simulink model "differential"  (R2018a)
settings: Solver=VariableStepDiscrete  StartTime=0.0  StopTime=0.15  RelTol=1e-3
undefined symbols (not defined in the file or in its folder): DiscIntNeverNeededParam
libraries: powerlib x45
settings Model: Creator=user  LastModifiedBy=user

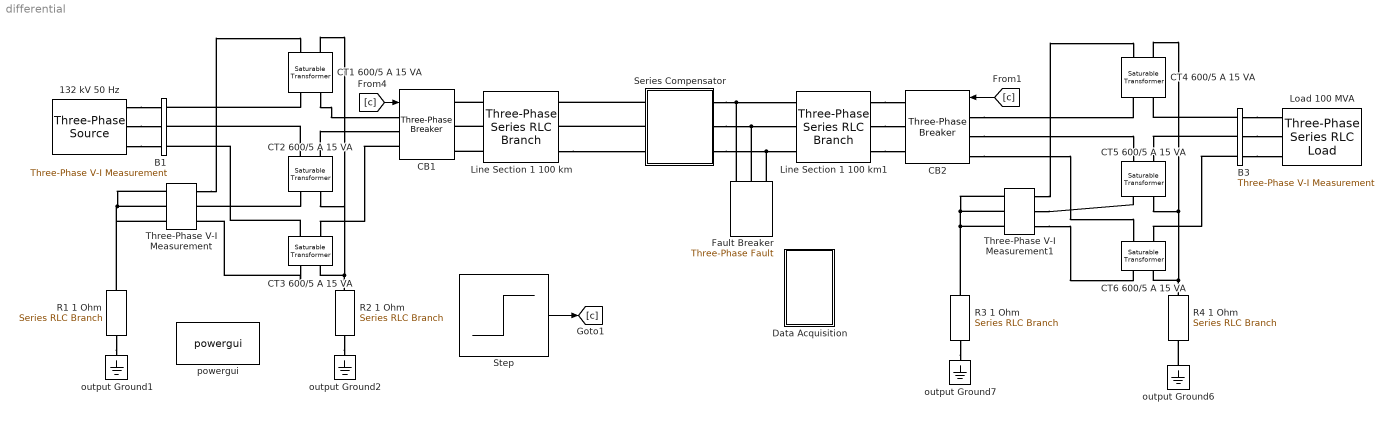
== system differential ==
  132 kV 50 Hz : powerlib/Electrical Sources/Three-Phase Source  InternalConnection=Yg  VoltagePhases=off  Voltage=132e3  PhaseAngle=0  Voltage_phases=[25e3 25e3 25e3]/sqrt(3)  PhaseAngles_phases=[0 -120 +120]  Frequency=50  NonIdealSource=on  SpecifyImpedance=on  Resistance=132^2/30000/10  Inductance=132^2/30000/377  ShortCircuitLevel=1000e6  BaseVoltage=132e3  XRratio=10  BusType=swing  Pref=150e6  Qref=0  Prefabc=[10e3, 10e3, 10e3]  Qrefabc=[0, 0, 0]  Qmin=0  Qmax=5e6
  B1 : powerlib/Measurements/Three-Phase V-I Measurement  VoltageMeasurement=phase-to-phase  SetLabelV=on  LabelV=Vabc_B1  Vpu=off  VpuLL=on  CurrentMeasurement=yes  SetLabelI=on  LabelI=Iabc_B1  Ipu=off  Pbase=100e6  Vbase=132e3  OutputType=Complex  PhasorSimulation=off  PSBequivalent=0
  B3 : powerlib/Measurements/Three-Phase V-I Measurement  VoltageMeasurement=phase-to-phase  SetLabelV=on  LabelV=Vabc_B2  Vpu=off  VpuLL=on  CurrentMeasurement=yes  SetLabelI=on  LabelI=Iabc_B2  Ipu=off  Pbase=100e6  Vbase=132e3  OutputType=Complex  PhasorSimulation=off  PSBequivalent=0
  CB1 : powerlib/Elements/Three-Phase Breaker  InitialState=closed  SwitchA=off  SwitchB=off  SwitchC=off  SwitchTimes=[5/60]  External=on  BreakerResistance=0.001  SnubberResistance=10e6  SnubberCapacitance=inf  Measurements=None
      settings: AttributesFormatString=\n
  CB2 : powerlib/Elements/Three-Phase Breaker  InitialState=closed  SwitchA=off  SwitchB=off  SwitchC=off  SwitchTimes=[5/60]  External=on  BreakerResistance=0.001  SnubberResistance=10e6  SnubberCapacitance=inf  Measurements=None
      settings: AttributesFormatString=\n
  CT1 600/5 A 15 VA : powerlib/Elements/Saturable Transformer  ThreeWindings=off  Hysteresis=off  DataFile='hysteresis'  Measurements=Winding currents  UNITS=pu  NominalPower=[15 50]  Winding1=[5*1/600 0.001 0.04]  Winding2=[5 0.001 0.04]  Winding3=[5 0.001 0.039999]  Saturation=[0 0 ; 0.01 10 ; 1 10.5]  CoreLoss=100  MoreParameters=off  BreakLoop=off  DataType=off  InitialFlux=-9.06091866417811e-08  TransfoNumber=1
      settings: AttributesFormatString=\n  SourceProductName=Simscape Power Systems  SourceProductBaseCode=PS
  CT2 600/5 A 15 VA : powerlib/Elements/Saturable Transformer  ThreeWindings=off  Hysteresis=off  DataFile='hysteresis'  Measurements=Winding currents  UNITS=pu  NominalPower=[15 50]  Winding1=[5*1/600 0.001 0.04]  Winding2=[5 0.001 0.04 ]  Winding3=[5 0.001 0.04 ]  Saturation=[0 0 ; 0.01 10 ; 1 10.5]  CoreLoss=100  MoreParameters=off  BreakLoop=off  DataType=off  InitialFlux=-1.84905677710759e-08  TransfoNumber=1
      settings: AttributesFormatString=\n  SourceProductName=Simscape Power Systems  SourceProductBaseCode=PS
  CT3 600/5 A 15 VA : powerlib/Elements/Saturable Transformer  ThreeWindings=off  Hysteresis=off  DataFile='hysteresis'  Measurements=Winding currents  UNITS=pu  NominalPower=[15 50]  Winding1=[5*1/600 0.001 0.04]  Winding2=[5 0.001 0.04]  Winding3=[5 0.001 0.039999]  Saturation=[0 0 ; 0.01 10 ; 1 10.5]  CoreLoss=100  MoreParameters=off  BreakLoop=off  DataType=off  InitialFlux=1.09099754414671e-07  TransfoNumber=1
      settings: AttributesFormatString=\n  SourceProductName=Simscape Power Systems  SourceProductBaseCode=PS
  CT4 600/5 A 15 VA : powerlib/Elements/Saturable Transformer  ThreeWindings=off  Hysteresis=off  DataFile='hysteresis'  Measurements=Winding currents  UNITS=pu  NominalPower=[15 50]  Winding1=[5*1/600 0.001 0.04]  Winding2=[5 0.001 0.04]  Winding3=[5 0.001 0.039999]  Saturation=[0 0 ; 0.01 10 ; 1 10.5]  CoreLoss=100  MoreParameters=off  BreakLoop=off  DataType=off  InitialFlux=-9.06015492379664e-08  TransfoNumber=1
      settings: AttributesFormatString=\n  SourceProductName=Simscape Power Systems  SourceProductBaseCode=PS
  CT5 600/5 A 15 VA : powerlib/Elements/Saturable Transformer  ThreeWindings=off  Hysteresis=off  DataFile='hysteresis'  Measurements=Winding currents  UNITS=pu  NominalPower=[15 50]  Winding1=[5*1/600 0.001 0.04]  Winding2=[5 0.001 0.04 ]  Winding3=[5 0.001 0.04 ]  Saturation=[0 0 ; 0.01 10 ; 1 10.5]  CoreLoss=100  MoreParameters=off  BreakLoop=off  DataType=off  InitialFlux=-1.84519480177304e-08  TransfoNumber=1
      settings: AttributesFormatString=\n  SourceProductName=Simscape Power Systems  SourceProductBaseCode=PS
  CT6 600/5 A 15 VA : powerlib/Elements/Saturable Transformer  ThreeWindings=off  Hysteresis=off  DataFile='hysteresis'  Measurements=Winding currents  UNITS=pu  NominalPower=[15 50]  Winding1=[5*1/600 0.001 0.04]  Winding2=[5 0.001 0.04]  Winding3=[5 0.001 0.039999]  Saturation=[0 0 ; 0.01 10 ; 1 10.5]  CoreLoss=100  MoreParameters=off  BreakLoop=off  DataType=off  InitialFlux=1.09053497257451e-07  TransfoNumber=1
      settings: AttributesFormatString=\n  SourceProductName=Simscape Power Systems  SourceProductBaseCode=PS
  Data Acquisition : Subsystem  mask(Data Acquisition){}
      mask Display: disp('Scopes')
  Fault Breaker : powerlib/Elements/Three-Phase Fault  InitialStates=0  FaultA=on  FaultB=off  FaultC=off  GroundFault=off  SwitchTimes=[2.5/60 ]  External=off  SwitchStatus=NaN  FaultResistance=0.001  GroundResistance=0.01  SnubberResistance=1e6  SnubberCapacitance=inf  Measurements=Fault currents
  Line Section 1 100 km : powerlib/Elements/Three-Phase Series RLC Branch  LConnTagsString=A|B|C  RConnTagsString=A|B|C  BranchType=RL  Resistance=36.7  Inductance=0.462  Capacitance=0.001  Measurements=None
  Line Section 1 100 km1 : powerlib/Elements/Three-Phase Series RLC Branch  LConnTagsString=A|B|C  RConnTagsString=A|B|C  BranchType=RL  Resistance=36.7  Inductance=0.462  Capacitance=0.001  Measurements=None
  Load 100 MVA : powerlib/Elements/Three-Phase Series RLC Load  LConnTagsString=A|B|C  Configuration=Y (grounded)  NominalVoltage=132e3  Vabc=[1e3 1e3 1e3]  Vabcp=[1e3 1e3 1e3]  NominalFrequency=50  UnbalancedPower=off  ActivePower=50e6  InductivePower=25e6  CapacitivePower=0  Pabc=[10e3 9e3 11e3]  QLabc=[100 90 110]  QCabc=[100 90 110]  Pabcp=[10e3 9e3 11e3]  QLabcp=[100 90 110]  QCabcp=[100 90 110]  Measurements=None  LoadType=constant Z
  R1 1 Ohm : powerlib/Elements/Series RLC Branch  LConnTagsString=__new0  RConnTagsString=__new0  BranchType=R  Resistance=1  Inductance=[]  SetiL0=off  InitialCurrent=0  Capacitance=[]  Setx0=off  InitialVoltage=0  Measurements=None
  R2 1 Ohm : powerlib/Elements/Series RLC Branch  LConnTagsString=__new0  RConnTagsString=__new0  BranchType=R  Resistance=1  Inductance=[]  SetiL0=off  InitialCurrent=0  Capacitance=[]  Setx0=off  InitialVoltage=0  Measurements=None
  R3 1 Ohm : powerlib/Elements/Series RLC Branch  LConnTagsString=__new0  RConnTagsString=__new0  BranchType=R  Resistance=1  Inductance=[]  SetiL0=off  InitialCurrent=0  Capacitance=[]  Setx0=off  InitialVoltage=0  Measurements=None
  R4 1 Ohm : powerlib/Elements/Series RLC Branch  LConnTagsString=__new0  RConnTagsString=__new0  BranchType=R  Resistance=1  Inductance=[]  SetiL0=off  InitialCurrent=0  Capacitance=[]  Setx0=off  InitialVoltage=0  Measurements=None
  Series Compensator : Subsystem
      mask Display: plot(0,0,100,100,[25 45],[50 50], [45 45],[35 65],[55 55],[35 65], [55 75],[50 50])
  Step : Step  Time=2/60  Before=1  VectorParams1D=off  ZeroCross=off
  Three-Phase V-I Measurement : powerlib/Measurements/Three-Phase V-I Measurement  VoltageMeasurement=no  SetLabelV=off  LabelV=Vabc  Vpu=off  VpuLL=off  CurrentMeasurement=yes  SetLabelI=on  LabelI=Iabc  Ipu=off  Pbase=100e6  Vbase=500e3  OutputType=Complex  PhasorSimulation=off  PSBequivalent=0
  Three-Phase V-I Measurement1 : powerlib/Measurements/Three-Phase V-I Measurement  VoltageMeasurement=no  SetLabelV=off  LabelV=Vabc  Vpu=off  VpuLL=off  CurrentMeasurement=yes  SetLabelI=on  LabelI=Iabc1  Ipu=off  Pbase=100e6  Vbase=500e3  OutputType=Complex  PhasorSimulation=off  PSBequivalent=0
  output Ground{1..2,6..7} (4 alike) : powerlib/Elements/Ground  LConnTagsString=a
  powergui : powerlib/powergui  Priority=2  SimulationMode=Discrete  SampleTime=50e-6  frequency=60  Iterations=50  frequencyindice=50  Pbase=100e6  ErrMax=0.0001  UnitsV=kV  UnitsW=MW  buscounter=0  FunctionMessages=off  echomessages=off  EnableUseOfTLC=off  CurrentSourceSwitches=off  DisableSnubberDevices=off  DisableRonSwitches=off  DisableVfSwitches=off  DisplayEquations=off  SolverType=Tustin/Backward Euler (TBE)  Interpol=off  ExternalGateDelay=off  methode=off  Ts=100  x0status=blocks  SPID=off  SwTol=0  HookPort=off  RestoreLinks=warning  ResistiveCurrentMeasurement=off  Frange=0:0.5:500  Ylog=off  Xlog=off  ShowGrid=off  save=on  variable=Zmes  structure=0  ZoomFFT=on  StartTime=0.0  cycles=1  DisplayStyle=off  fundamental=60  FreqAxis=off  MaxFrequency=1000  frequencyindicesteady=1  RmsSteady=1  display=off
  wires:
  [c] -> CB1/1
  [c] -> CB2/1
  Step/1 -> [c]
  connections:
  Three-Phase V-I Measurement/RConn2 -- Three-Phase V-I Measurement/RConn1 -- R1 1 Ohm/LConn1 -- Three-Phase V-I Measurement/RConn3
  R2 1 Ohm/LConn1 -- CT1 600/5 A 15 VA/RConn2 -- CT2 600/5 A 15 VA/RConn2 -- CT3 600/5 A 15 VA/RConn2
  Series Compensator/RConn3 -- Line Section 1 100 km1/LConn3 -- Fault Breaker/LConn3
  Series Compensator/RConn2 -- Line Section 1 100 km1/LConn2 -- Fault Breaker/LConn2
  Series Compensator/RConn1 -- Line Section 1 100 km1/LConn1 -- Fault Breaker/LConn1
  R1 1 Ohm/RConn1 -- output Ground1/LConn1
  Line Section 1 100 km/LConn2 -- CB1/RConn2
  CT2 600/5 A 15 VA/RConn1 -- Three-Phase V-I Measurement/LConn2
  CT3 600/5 A 15 VA/RConn1 -- Three-Phase V-I Measurement/LConn3
  Three-Phase V-I Measurement/LConn1 -- CT1 600/5 A 15 VA/RConn1
  CT1 600/5 A 15 VA/LConn2 -- CB1/LConn1
  Line Section 1 100 km/RConn3 -- Series Compensator/LConn3
  CT2 600/5 A 15 VA/LConn1 -- B1/RConn2
  R2 1 Ohm/RConn1 -- output Ground2/LConn1
  Line Section 1 100 km/LConn3 -- CB1/RConn3
  132 kV 50 Hz/RConn1 -- B1/LConn1
  Series Compensator/LConn2 -- Line Section 1 100 km/RConn2
  Series Compensator/LConn1 -- Line Section 1 100 km/RConn1
  CB1/LConn3 -- CT3 600/5 A 15 VA/LConn2
  CT1 600/5 A 15 VA/LConn1 -- B1/RConn1
  132 kV 50 Hz/RConn2 -- B1/LConn2
  Line Section 1 100 km/LConn1 -- CB1/RConn1
  CT3 600/5 A 15 VA/LConn1 -- B1/RConn3
  132 kV 50 Hz/RConn3 -- B1/LConn3
  CT2 600/5 A 15 VA/LConn2 -- CB1/LConn2
  CT5 600/5 A 15 VA/RConn2 -- CT4 600/5 A 15 VA/RConn2 -- R4 1 Ohm/LConn1 -- CT6 600/5 A 15 VA/RConn2
  Three-Phase V-I Measurement1/RConn3 -- R3 1 Ohm/LConn1 -- Three-Phase V-I Measurement1/RConn2 -- Three-Phase V-I Measurement1/RConn1
  B3/RConn3 -- Load 100 MVA/LConn3
  B3/LConn3 -- CT6 600/5 A 15 VA/LConn2
  Line Section 1 100 km1/RConn1 -- CB2/RConn1
  output Ground6/LConn1 -- R4 1 Ohm/RConn1
  Line Section 1 100 km1/RConn2 -- CB2/RConn2
  R3 1 Ohm/RConn1 -- output Ground7/LConn1
  CB2/LConn1 -- CT4 600/5 A 15 VA/LConn1
  CB2/LConn2 -- CT5 600/5 A 15 VA/LConn1
  Three-Phase V-I Measurement1/LConn2 -- CT5 600/5 A 15 VA/RConn1
  Three-Phase V-I Measurement1/LConn1 -- CT4 600/5 A 15 VA/RConn1
  B3/LConn2 -- CT5 600/5 A 15 VA/LConn2
  B3/LConn1 -- CT4 600/5 A 15 VA/LConn2
  CB2/LConn3 -- CT6 600/5 A 15 VA/LConn1
  Line Section 1 100 km1/RConn3 -- CB2/RConn3
  B3/RConn1 -- Load 100 MVA/LConn1
  B3/RConn2 -- Load 100 MVA/LConn2
  Three-Phase V-I Measurement1/LConn3 -- CT6 600/5 A 15 VA/RConn1

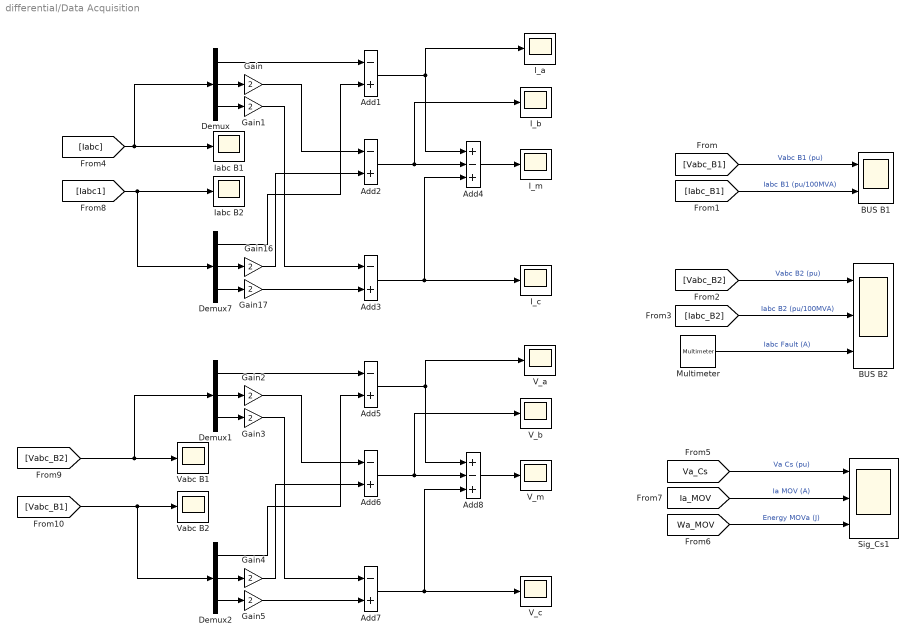
== system differential/Data Acquisition ==
  Add{1..3,5..7} (6 alike) : Sum  Inputs=-+
  Add4 : Sum  Inputs=+-+
  Add8 : Sum  Inputs=+-+
  BUS B1 : Scope  NumInputPorts=2
  BUS B2 : Scope  NumInputPorts=3
  Demux{,1..2,7} (4 alike) : Demux  Outputs=3
  Gain{,1..5,16..17} (8 alike) : Gain  Gain=2
  I_a : Scope
  I_b : Scope
  I_c : Scope
  I_m : Scope
  Iabc B1 : Scope
  Iabc B2 : Scope
  Multimeter : powerlib/Measurements/Multimeter  Tag=PoWeRsYsTeMmEaSuReMeNt  PhasorSimulation=off  OutputType=Magnitude  sel=[1 2 3]  L=15  Gain=[1 1 1]  yselected={'Ib: Fault Breaker/Fault A','Ib: Fault Breaker/Fault B','Ib: Fault Breaker/Fault C'};  PSBOutputType=1  PSBequivalent=0  AxesSetting=[0,0.1,-100,100]  Display=0  SavedBlockNames={}
      settings: AttributesFormatString=\n
  Sig_Cs1 : Scope  NumInputPorts=3
  V_a : Scope
  V_b : Scope
  V_c : Scope
  V_m : Scope
  Vabc B1 : Scope
  Vabc B2 : Scope
  wires:
  [Vabc_B1] -> BUS B1/1  "Vabc B1 (pu)"
  [Iabc_B1] -> BUS B1/2  "Iabc B1 (pu/100MVA)"
  [Vabc_B2] -> BUS B2/1  "Vabc B2 (pu)"
  [Iabc_B2] -> BUS B2/2  "Iabc B2 (pu/100MVA)"
  [Va_Cs] -> Sig_Cs1/1  "Va Cs (pu)"
  [Ia_MOV] -> Sig_Cs1/2  "Ia MOV (A)"
  [Wa_MOV] -> Sig_Cs1/3  "Energy MOVa (J)"
  Multimeter/1 -> BUS B2/3  "Iabc Fault (A)"
  Gain/1 -> Add2/1
  Demux/3 -> Gain1/1
  Demux/2 -> Gain/1
  Gain1/1 -> Add3/1
  [Iabc] -> Iabc B1/1, Demux/1
  [Iabc1] -> Iabc B2/1, Demux7/1
  Gain17/1 -> Add3/2
  Demux7/3 -> Gain17/1
  Demux7/1 -> Add1/2
  Demux7/2 -> Gain16/1
  Demux/1 -> Add1/1
  Gain16/1 -> Add2/2
  Add4/1 -> I_m/1
  Add1/1 -> I_a/1, Add4/1
  Add2/1 -> I_b/1, Add4/2
  Add3/1 -> Add4/3, I_c/1
  Demux2/3 -> Gain5/1
  Demux1/1 -> Add5/1
  [Vabc_B1] -> Vabc B2/1, Demux2/1
  [Vabc_B2] -> Vabc B1/1, Demux1/1
  Add8/1 -> V_m/1
  Gain4/1 -> Add6/2
  Gain2/1 -> Add6/1
  Gain5/1 -> Add7/2
  Add6/1 -> V_b/1, Add8/2
  Demux1/3 -> Gain3/1
  Demux1/2 -> Gain2/1
  Demux2/1 -> Add5/2
  Gain3/1 -> Add7/1
  Add5/1 -> V_a/1, Add8/1
  Demux2/2 -> Gain4/1
  Add7/1 -> Add8/3, V_c/1

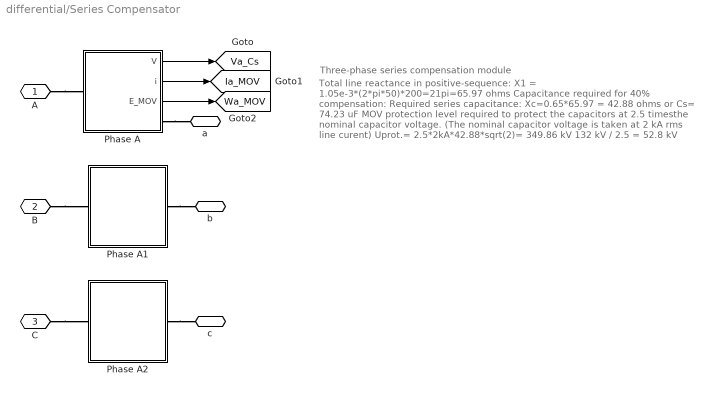
== system differential/Series Compensator ==
  note: Three-phase series compensation module
  note: Total line reactance in positive-sequence:
      |  X1 = 1.05e-3*(2*pi*50)*200=21pi=65.97 ohms
      |
      | Capacitance required for 40% compensation:
      |
      | Required series capacitance:
      | Xc=0.65*65.97 = 42.88 ohms
      | or Cs= 74.23 uF
      |
      | MOV protection level required to protect the capacitors
      | at 2.5 timesthe nominal capacitor voltage.
      | (The nominal capacitor voltage is taken at 2 kA  rms line curent)
      |
      | Uprot.= 2.5*2kA*42.88*sqrt(2)= 349.86 kV
      |
      | 132 kV / 2.5 = 52.8 kV
  Phase A : Subsystem
  Phase A1 : Subsystem
  Phase A2 : Subsystem
  A : PMIOPort  Side=Left
  B : PMIOPort  Port=2  Side=Left
  C : PMIOPort  Port=3  Side=Left
  a : PMIOPort  Port=4  Side=Right
  b : PMIOPort  Port=5  Side=Right
  c : PMIOPort  Port=6  Side=Right
  tag scope: Ia_MOV=global, Va_Cs=global, Wa_MOV=global
  wires:
  Phase A/2(i) -> [Ia_MOV]
  Phase A/1(V) -> [Va_Cs]
  Phase A/3(E_MOV) -> [Wa_MOV]
  connections:
  A/RConn1 -- Phase A/LConn1
  B/RConn1 -- Phase A1/LConn1
  C/RConn1 -- Phase A2/LConn1
  Phase A/RConn1 -- a/RConn1
  Phase A1/RConn1 -- b/RConn1
  Phase A2/RConn1 -- c/RConn1

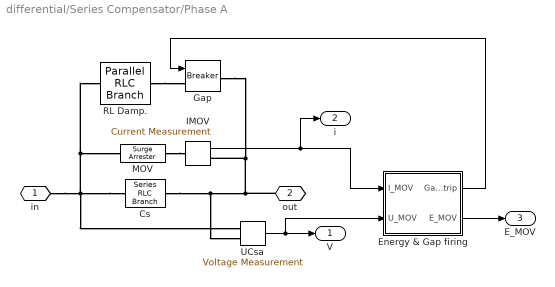
== system differential/Series Compensator/Phase A ==
  Cs : powerlib/Elements/Series RLC Branch  LConnTagsString=__new0  RConnTagsString=__new0  BranchType=C  Resistance=1.0  Inductance=1.0  SetiL0=off  InitialCurrent=0  Capacitance=95e-6  Setx0=off  InitialVoltage=0  Measurements=None
  Energy & Gap firing : Subsystem
  Gap : powerlib/Elements/Breaker  InitialState=0  SwitchingTimes="[ 4/60  5/60 ]"  External=on  BreakerResistance=0.001  SnubberResistance=inf  SnubberCapacitance=0  Measurements=None  MoreParameters=off  NoBreakLoop=off
      settings: AttributesFormatString=\n  SourceProductName=Simscape Power Systems
  IMOV : powerlib/Measurements/Current Measurement  Tag=PoWeRsYsTeMmEaSuReMeNt  PhasorSimulation=off  OutputType=Magnitude  PSBequivalent=0
  MOV : powerlib/Elements/Surge Arrester  ProtectionVoltage=54e+03  Columns=27  ReferenceCurrent=200  Segment1=[.955 50]  Segment2=[1.0 25]  Segment3=[.9915 16.5]  Measurements=None  BreakLoop=on
      settings: AttributesFormatString=\n  SourceProductName=Simscape Power Systems  SourceProductBaseCode=PS
  RL Damp. : powerlib/Elements/Parallel RLC Branch  LConnTagsString=a  RConnTagsString=__new0  BranchType=RL  Resistance=7.5  Inductance=1.7e-3  SetiL0=off  InitialCurrent=0  Capacitance=1.0  Setx0=off  InitialVoltage=0  Measurements=None
  UCsa : powerlib/Measurements/Voltage Measurement  Tag=PoWeRsYsTeMmEaSuReMeNt  PhasorSimulation=off  OutputType=Magnitude  PSBequivalent=0
  in : PMIOPort  Side=Left
  "out " : PMIOPort  Port=2  Side=Right
  V : Outport
  i : Outport  Port=2
  E_MOV : Outport  Port=3
  wires:
  Energy & Gap firing/2(E_MOV) -> E_MOV/1
  IMOV/1 -> Energy & Gap firing/1(I_MOV), i/1
  UCsa/1 -> Energy & Gap firing/2(U_MOV), V/1
  Energy & Gap firing/1(Gap_trip) -> Gap/1
  connections:
  MOV/RConn1 -- IMOV/LConn1
  Cs/LConn1 -- UCsa/LConn1 -- in/RConn1 -- RL Damp./LConn1 -- MOV/LConn1
  RL Damp./RConn1 -- Gap/LConn1
  Cs/RConn1 -- "out "/RConn1 -- IMOV/RConn1 -- Gap/RConn1 -- UCsa/LConn2

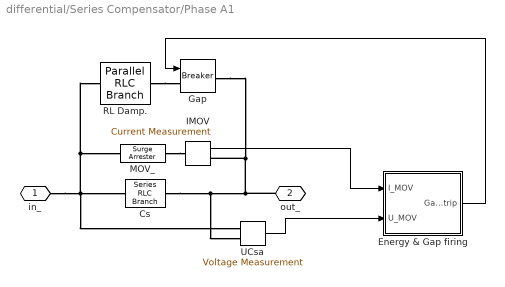
== system differential/Series Compensator/Phase A1 ==
  Cs : powerlib/Elements/Series RLC Branch  LConnTagsString=__new0  RConnTagsString=__new0  BranchType=C  Resistance=1.0  Inductance=1.0  SetiL0=off  InitialCurrent=0  Capacitance=95e-6  Setx0=off  InitialVoltage=0  Measurements=None
  Energy & Gap firing : Subsystem
  Gap : powerlib/Elements/Breaker  InitialState=0  SwitchingTimes="[ 4/60  5/60 ]"  External=on  BreakerResistance=0.001  SnubberResistance=inf  SnubberCapacitance=0  Measurements=None  MoreParameters=off  NoBreakLoop=off
      settings: AttributesFormatString=\n  SourceProductName=Simscape Power Systems
  IMOV : powerlib/Measurements/Current Measurement  Tag=PoWeRsYsTeMmEaSuReMeNt  PhasorSimulation=off  OutputType=Magnitude  PSBequivalent=0
  MOV_ : powerlib/Elements/Surge Arrester  ProtectionVoltage=54e+03  Columns=27  ReferenceCurrent=200  Segment1=[.955 50]  Segment2=[1.0 25]  Segment3=[.9915 16.5]  Measurements=None  BreakLoop=on
      settings: AttributesFormatString=\n  SourceProductName=Simscape Power Systems  SourceProductBaseCode=PS
  RL Damp. : powerlib/Elements/Parallel RLC Branch  LConnTagsString=a  RConnTagsString=__new0  BranchType=RL  Resistance=7.5  Inductance=1.7e-3  SetiL0=off  InitialCurrent=0  Capacitance=1.0  Setx0=off  InitialVoltage=0  Measurements=None
  UCsa : powerlib/Measurements/Voltage Measurement  Tag=PoWeRsYsTeMmEaSuReMeNt  PhasorSimulation=off  OutputType=Magnitude  PSBequivalent=0
  in_ : PMIOPort  Side=Left
  "out_ " : PMIOPort  Port=2  Side=Right
  wires:
  Energy & Gap firing/1(Gap_trip) -> Gap/1
  UCsa/1 -> Energy & Gap firing/2(U_MOV)
  IMOV/1 -> Energy & Gap firing/1(I_MOV)
  connections:
  "out_ "/RConn1 -- UCsa/LConn2 -- Cs/RConn1 -- Gap/RConn1 -- IMOV/RConn1
  RL Damp./RConn1 -- Gap/LConn1
  in_/RConn1 -- UCsa/LConn1 -- Cs/LConn1 -- MOV_/LConn1 -- RL Damp./LConn1
  MOV_/RConn1 -- IMOV/LConn1

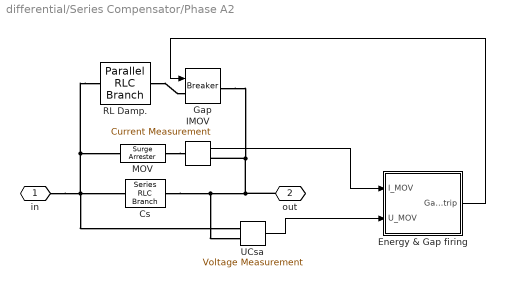
== system differential/Series Compensator/Phase A2 ==
  Cs : powerlib/Elements/Series RLC Branch  LConnTagsString=__new0  RConnTagsString=__new0  BranchType=C  Resistance=1.0  Inductance=1.0  SetiL0=off  InitialCurrent=0  Capacitance=95e-6  Setx0=off  InitialVoltage=0  Measurements=None
  Energy & Gap firing : Subsystem
  Gap : powerlib/Elements/Breaker  InitialState=0  SwitchingTimes="[ 4/60  5/60 ]"  External=on  BreakerResistance=0.001  SnubberResistance=inf  SnubberCapacitance=0  Measurements=None  MoreParameters=off  NoBreakLoop=off
      settings: AttributesFormatString=\n  SourceProductName=Simscape Power Systems
  IMOV : powerlib/Measurements/Current Measurement  Tag=PoWeRsYsTeMmEaSuReMeNt  PhasorSimulation=off  OutputType=Magnitude  PSBequivalent=0
  MOV : powerlib/Elements/Surge Arrester  ProtectionVoltage=54e+03  Columns=27  ReferenceCurrent=200  Segment1=[.955 50]  Segment2=[1.0 25]  Segment3=[.9915 16.5]  Measurements=None  BreakLoop=on
      settings: AttributesFormatString=\n  SourceProductName=Simscape Power Systems  SourceProductBaseCode=PS
  RL Damp. : powerlib/Elements/Parallel RLC Branch  LConnTagsString=a  RConnTagsString=__new0  BranchType=RL  Resistance=7.5  Inductance=1.7e-3  SetiL0=off  InitialCurrent=0  Capacitance=1.0  Setx0=off  InitialVoltage=0  Measurements=None
  UCsa : powerlib/Measurements/Voltage Measurement  Tag=PoWeRsYsTeMmEaSuReMeNt  PhasorSimulation=off  OutputType=Magnitude  PSBequivalent=0
  in : PMIOPort  Side=Left
  "out " : PMIOPort  Port=2  Side=Right
  wires:
  IMOV/1 -> Energy & Gap firing/1(I_MOV)
  UCsa/1 -> Energy & Gap firing/2(U_MOV)
  Energy & Gap firing/1(Gap_trip) -> Gap/1
  connections:
  MOV/RConn1 -- IMOV/LConn1
  RL Damp./LConn1 -- MOV/LConn1 -- Cs/LConn1 -- UCsa/LConn1 -- in/RConn1
  RL Damp./RConn1 -- Gap/LConn1
  IMOV/RConn1 -- Gap/RConn1 -- Cs/RConn1 -- UCsa/LConn2 -- "out "/RConn1

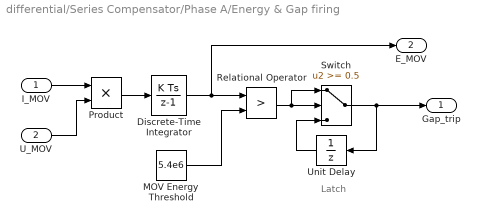
== system differential/Series Compensator/Phase A/Energy & Gap firing ==
  note: Latch
  I_MOV : Inport
  U_MOV : Inport  Port=2
  Discrete-Time Integrator : DiscreteIntegrator  SampleTime=-1  ICPrevOutput=DiscIntNeverNeededParam  ICPrevScaledInput=DiscIntNeverNeededParam
  MOV Energy Threshold : Constant  Value=5.4e6
  Product : Product  SaturateOnIntegerOverflow=on  InputSameDT=on  OutDataTypeStr=Inherit: Same as first input
  Relational Operator : RelationalOperator  Operator=>  ZeroCross=off  RndMeth=Nearest  InputSameDT=on
  Switch : Switch  Threshold=0.5  ZeroCross=off  InputSameDT=on
  Unit Delay : UnitDelay  SampleTime=-1
  Gap_trip : Outport
  E_MOV : Outport  Port=2  InitialOutput=0
  wires:
  Switch/1 -> Unit Delay/1, Gap_trip/1
  U_MOV/1 -> Product/2
  MOV Energy Threshold/1 -> Relational Operator/2
  Product/1 -> Discrete-Time Integrator/1
  I_MOV/1 -> Product/1
  Discrete-Time Integrator/1 -> E_MOV/1, Relational Operator/1
  Relational Operator/1 -> Switch/1, Switch/2
  Unit Delay/1 -> Switch/3

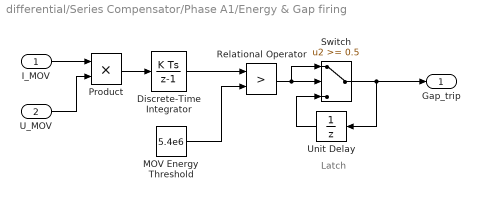
== system differential/Series Compensator/Phase A1/Energy & Gap firing ==
  note: Latch
  I_MOV : Inport
  U_MOV : Inport  Port=2
  Discrete-Time Integrator : DiscreteIntegrator  SampleTime=-1  ICPrevOutput=DiscIntNeverNeededParam  ICPrevScaledInput=DiscIntNeverNeededParam
  MOV Energy Threshold : Constant  Value=5.4e6
  Product : Product  SaturateOnIntegerOverflow=on  InputSameDT=on  OutDataTypeStr=Inherit: Same as first input
  Relational Operator : RelationalOperator  Operator=>  ZeroCross=off  RndMeth=Nearest  InputSameDT=on
  Switch : Switch  Threshold=0.5  ZeroCross=off  InputSameDT=on
  Unit Delay : UnitDelay  SampleTime=-1
  Gap_trip : Outport
  wires:
  Unit Delay/1 -> Switch/3
  Relational Operator/1 -> Switch/2, Switch/1
  Discrete-Time Integrator/1 -> Relational Operator/1
  I_MOV/1 -> Product/1
  Product/1 -> Discrete-Time Integrator/1
  MOV Energy Threshold/1 -> Relational Operator/2
  U_MOV/1 -> Product/2
  Switch/1 -> Gap_trip/1, Unit Delay/1

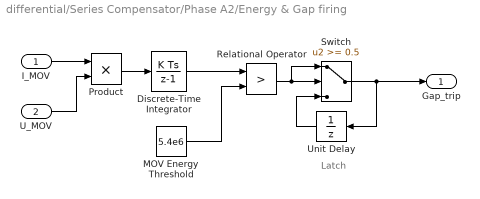
== system differential/Series Compensator/Phase A2/Energy & Gap firing ==
  note: Latch
  I_MOV : Inport
  U_MOV : Inport  Port=2
  Discrete-Time Integrator : DiscreteIntegrator  SampleTime=-1  ICPrevOutput=DiscIntNeverNeededParam  ICPrevScaledInput=DiscIntNeverNeededParam
  MOV Energy Threshold : Constant  Value=5.4e6
  Product : Product  SaturateOnIntegerOverflow=on  InputSameDT=on  OutDataTypeStr=Inherit: Same as first input
  Relational Operator : RelationalOperator  Operator=>  ZeroCross=off  RndMeth=Nearest  InputSameDT=on
  Switch : Switch  Threshold=0.5  ZeroCross=off  InputSameDT=on
  Unit Delay : UnitDelay  SampleTime=-1
  Gap_trip : Outport
  wires:
  Switch/1 -> Unit Delay/1, Gap_trip/1
  U_MOV/1 -> Product/2
  MOV Energy Threshold/1 -> Relational Operator/2
  Product/1 -> Discrete-Time Integrator/1
  I_MOV/1 -> Product/1
  Discrete-Time Integrator/1 -> Relational Operator/1
  Relational Operator/1 -> Switch/1, Switch/2
  Unit Delay/1 -> Switch/3
